simulink model "delayerror2"  (Simulink 6.4)
settings: Solver=ode4  SolverMode=SingleTasking  StartTime=0.0  StopTime=10.0  FixedStep=0.001  RelTol=1e-3  AbsTol=1e-6
settings Model: Creator=jacobs  LastModifiedBy=jacobs  ExtModeAutoUpdateStatusClock=off
settings DataIOCC: LimitDataPoints=off
settings OptimizationCC: BlockReduction=off  BooleanDataType=off
settings DebuggingCC: SolverPrmCheckMsg=none  UnconnectedInputMsg=none  UnconnectedOutputMsg=none  StrictBusMsg=None
settings HardwareCC: TargetUnknown=on
settings GRTTargetCC: ModelReferenceCompliant=off  MatFileLogging=off

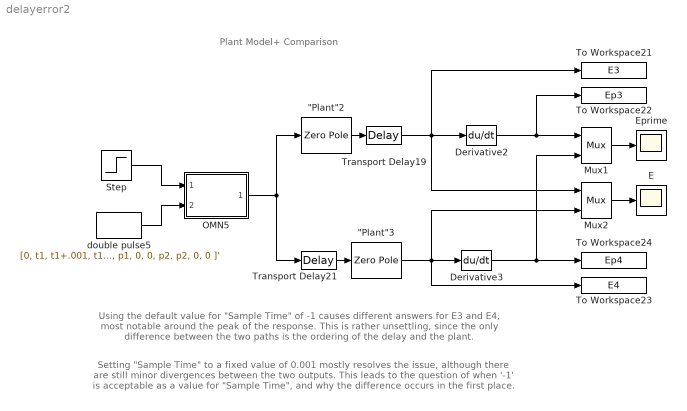
== system delayerror2 ==
  note: Plant Model+ Comparison
  note: Using the default value for "Sample Time" of -1 causes different answers for E3 and E4, most notable
      | around the peak of the response.  This is rather unsettling, since the only difference between the two
      | paths is the ordering of the delay and the plant.
  note: Setting "Sample Time" to a fixed value of 0.001 mostly resolves the issue, although there are still minor
      | divergences between the two outputs.  This leads to the question of when '-1' is acceptable as a value
      | for "Sample Time", and why the difference occurs in the first place.
  "\"Plant\"2" : ZeroPole  Zeros=[ ]  Poles=[ -1/.18 -1/.007]  Gain=[1/.18 * 1/.007]
      mask Display: disp('2-pole\n"Plant"')
  "\"Plant\"3" : ZeroPole  Zeros=[ ]  Poles=[ -1/.18 -1/.007]  Gain=[1/.18 * 1/.007]
      mask Display: disp('2-pole\n"Plant"')
  Derivative2 : Derivative
      mask Display: disp('s')
  Derivative3 : Derivative
      mask Display: disp('s')
  E : Scope
      settings: TickLabels=on  TimeRange=10  YMin=0  YMax=20  DataFormat=Array
  Eprime : Scope
      settings: TickLabels=on  TimeRange=10  YMin=-100  YMax=600  DataFormat=Array
  Mux1 : Mux  Inputs=2
  Mux2 : Mux  Inputs=2
  OMN5 : Subsystem
      mask Display: disp('<--tonic\nOMN2\n<--phasic')
  Step : Step  Time=2  After=15
  To Workspace21 : ToWorkspace  VariableName=E3  SaveFormat=Array
      settings: MaxDataPoints=10000
  To Workspace22 : ToWorkspace  VariableName=Ep3  SaveFormat=Array
      settings: MaxDataPoints=10000
  To Workspace23 : ToWorkspace  VariableName=E4  SaveFormat=Array
      settings: MaxDataPoints=10000
  To Workspace24 : ToWorkspace  VariableName=Ep4  SaveFormat=Array
      settings: MaxDataPoints=10000
  Transport Delay19 : TransportDelay  DelayTime=0.080
      mask Display: disp('80ms')
  Transport Delay21 : TransportDelay  DelayTime=0.080
      mask Display: disp('80ms')
  double pulse5 : FromWorkspace  VariableName=[0, t1, t1+.001, t1+d1, t1+d1+.001, t1+d1+.001+ipd, t1+d1+.001+ipd, t1+d1+.001+ipd+d2, t1+d1+.001+ipd+d2, 10000; 0, 0, p1, p1, 0, 0, p2, p2, 0, 0 ]'  mask{@1=96.25, @2=2, @3=0.031, @4=0, @5=0, @6=0}
      mask prompts: @1 "Pulse 1 Magnitude"; @2 "Time of Pulse 1 Onset"; @3 "Pulse 1 Duration"; @4 "Interpulse Delay"; @5 "Pulse 2 Magnitude"; @6 "Pulse 2 Duration"
      mask help: Double Pulse
      mask init:
      | p1=@1; t1=@2; d1=@3; ipd=@4; p2=@5; d2=@6;
      mask Display: disp('Double\nPulse')
  wires:
  Transport Delay21/1 -> "\"Plant\"3"/1
  Step/1 -> OMN5/1("[epossp]")
  double pulse5/1 -> OMN5/2("[pgout]")
  "\"Plant\"2"/1 -> Transport Delay19/1
  Transport Delay19/1 -> Derivative2/1, To Workspace21/1, Mux2/1
  "\"Plant\"3"/1 -> Derivative3/1, To Workspace23/1, Mux2/2
  Mux1/1 -> Eprime/1
  Derivative2/1 -> To Workspace22/1, Mux1/1
  Derivative3/1 -> To Workspace24/1, Mux1/2
  Mux2/1 -> E/1
  OMN5/1(out_1) -> "\"Plant\"2"/1, Transport Delay21/1

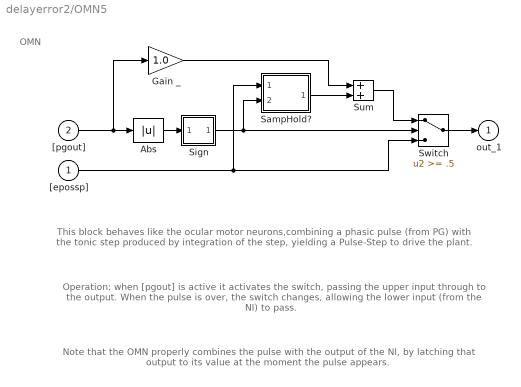
== system delayerror2/OMN5 ==
  note: OMN
  note: Note that the OMN properly combines the pulse with the output of the NI, by latching
      | that output to its value at the moment the pulse appears.
  note: Operation: when [pgout] is active it activates the switch, passing the
      | upper input through to the output.  When the pulse is over, the switch changes,
      | allowing the lower input (from the NI) to pass.
  note: This block behaves like the ocular motor neurons,combining a phasic pulse (from PG)
      | with the tonic step produced by integration of the step, yielding a Pulse-Step
      | to drive the plant.
  "[epossp]" : Inport
  "[pgout]" : Inport  Port=2
  Abs : Abs  SaturateOnIntegerOverflow=on
  Gain _ : Gain  Gain=1.0  SaturateOnIntegerOverflow=on
  SampHold? : Subsystem
      mask Display: disp('S=L\nH=H')
  Sign : Subsystem
      mask Type: Sign
      mask Description: y = sign(x)
      mask Help: Sign Function:\n\t\t\ty = 1 if x > 0\n\t\t\ty = 0 if x = 0\n\t\t\ty = -1 if x < 0
      mask Display: plot(-50,-50,50,50,[-50,50],[0,0],[0,0],[-50,50],[-40,0],[-30,-30],[0,40],[30,30])
  Sum : Sum  SaturateOnIntegerOverflow=on  InputSameDT=on
  Switch : Switch  Threshold=.5  SaturateOnIntegerOverflow=on  InputSameDT=on
  out_1 : Outport  InitialOutput=0
  wires:
  "[epossp]"/1 -> Switch/3, SampHold?/1(Input)
  Sign/1(out_1) -> Switch/2, SampHold?/2(S/H?)
  Gain _/1 -> Sum/1
  SampHold?/1(output) -> Sum/2
  Sum/1 -> Switch/1
  "[pgout]"/1 -> Abs/1, Gain _/1
  Switch/1 -> out_1/1
  Abs/1 -> Sign/1(in_1)

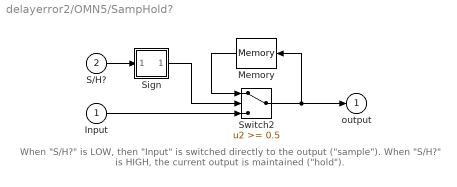
== system delayerror2/OMN5/SampHold? ==
  note: When "S/H?" is LOW, then "Input" is switched directly to the
      | output ("sample").  When "S/H?" is HIGH, the current output is
      | maintained ("hold").
  Input : Inport
  S/H? : Inport  Port=2
  Memory : Memory  Orientation=left
  Sign : Subsystem
      mask Type: Sign
      mask Description: y = sign(x)
      mask Help: Sign Function:\n\t\t\ty = 1 if x > 0\n\t\t\ty = 0 if x = 0\n\t\t\ty = -1 if x < 0
      mask Display: plot(-50,-50,50,50,[-50,50],[0,0],[0,0],[-50,50],[-40,0],[-30,-30],[0,40],[30,30])
  Switch2 : Switch  Threshold=0.5  SaturateOnIntegerOverflow=on  InputSameDT=on
  output : Outport  InitialOutput=0
  wires:
  Switch2/1 -> Memory/1, output/1
  Sign/1(out_1) -> Switch2/2
  Input/1 -> Switch2/3
  S/H?/1 -> Sign/1(in_1)
  Memory/1 -> Switch2/1

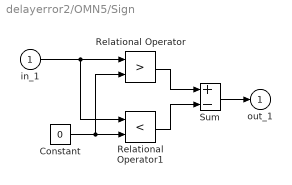
== system delayerror2/OMN5/Sign ==
  in_1 : Inport
  Constant : Constant  Value=0
  Relational Operator : RelationalOperator  Operator=>  InputSameDT=on
  Relational Operator1 : RelationalOperator  Operator=<  InputSameDT=on
  Sum : Sum  Inputs=+-  SaturateOnIntegerOverflow=on  InputSameDT=on
  out_1 : Outport  InitialOutput=0
  wires:
  Sum/1 -> out_1/1
  Relational Operator/1 -> Sum/1
  Relational Operator1/1 -> Sum/2
  Constant/1 -> Relational Operator1/2, Relational Operator/2
  in_1/1 -> Relational Operator/1, Relational Operator1/1

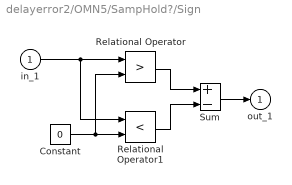
== system delayerror2/OMN5/SampHold?/Sign ==
  in_1 : Inport
  Constant : Constant  Value=0
  Relational Operator : RelationalOperator  Operator=>  InputSameDT=on
  Relational Operator1 : RelationalOperator  Operator=<  InputSameDT=on
  Sum : Sum  Inputs=+-  SaturateOnIntegerOverflow=on  InputSameDT=on
  out_1 : Outport  InitialOutput=0
  wires:
  in_1/1 -> Relational Operator/1, Relational Operator1/1
  Constant/1 -> Relational Operator1/2, Relational Operator/2
  Relational Operator1/1 -> Sum/2
  Relational Operator/1 -> Sum/1
  Sum/1 -> out_1/1
